simulink model "sysgenADCDAC"  (Simulink 7.3)
settings: Solver=ode45  StartTime=0.0  StopTime=20000  RelTol=1e-3
PreLoadFcn:
  | xlrequire('PreLoadFcn')
values from neighbouring files (symbols this model uses):
  Fstm = 0    [sysgenADCDAC_PreLoadFcn.m]
libraries: xbsIndex_r4 x94, xbsCopyrightNotice_r4 x1
settings Model: Creator=alexc  LastModifiedBy=douangp
settings DataIOCC: SignalLoggingName=sigsOut
settings OptimizationCC: BlockReduction=off  BooleanDataType=off  InlineInvariantSignals=on  InitFltsAndDblsToZero=on
settings DebuggingCC: SaveWithParameterizedLinksMsg=none  SignalResolutionControl=TryResolveAllWithWarning  SolverPrmCheckMsg=none  MultiTaskDSMMsg=warning  MultiTaskCondExecSysMsg=none  StrictBusMsg=None
settings HardwareCC: TargetUnknown=on
settings RTWCC: IncludeERTFirstTime=on
settings GRTTargetCC: TargetFcnLib=ansi_tfl_tmw.mat

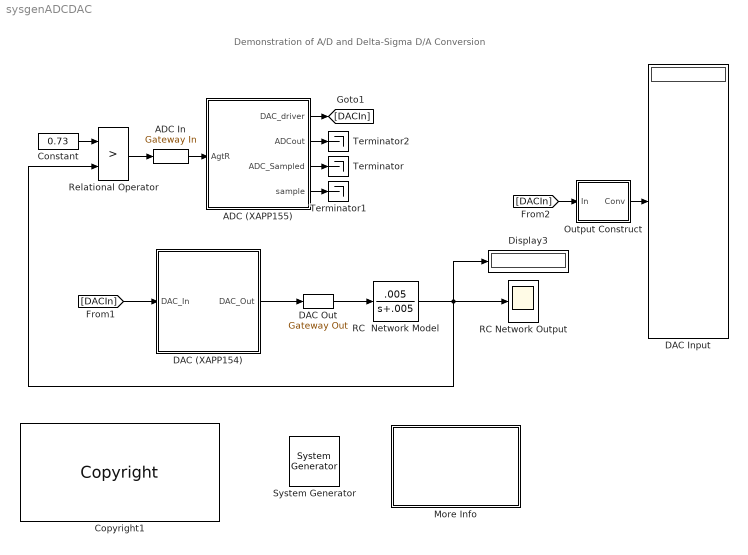
== system sysgenADCDAC ==
  note: Demonstration of A/D and Delta-Sigma D/A
      | Conversion
  " System Generator" : xbsIndex_r4/ System Generator  Tag=genX  SystemSampleTime=-1  xilinxfamily=virtex6  part=xc6vlx240t  speed=-1  package=ff1156  synthesis_tool=XST  clock_wrapper=Clock Enables  directory=./netlist  testbench=on  simulink_period=1  sysclk_period=2.5  dcm_input_clock_period=100  incr_netlist=off  trim_vbits=Everywhere in SubSystem  dbl_ovrd=According to Block Masks  core_generation=According to Block Masks  run_coregen=off  deprecated_control=off  eval_field=0  block_type=sysgen
      settings: block_version=9.2.00
  ADC (XAPP155) : Subsystem
  ADC In : xbsIndex_r4/Gateway In  arith_type=Unsigned  n_bits=1  bin_pt=0  quantization="Round  (unbiased: +/- Inf)"  overflow=Saturate  period=1  dbl_ovrd=off  timing_constraint=None  locs_specified=off  LOCs={}  block_type=gatewayin
      settings: infoedit="Gateway in block.  Converts inputs of type Simulink integer, double and fixed point to  Xilinx fixed point type.<P><P>Hardware notes:  In hardware these blocks become top level input ports."  xl_area=[0 0 0 0 1 0 0]  block_version=VER_STRING_GOES_HERE
  Constant : Constant  Value=0.73  OutDataType=sfix(16)  OutScaling=2^0
  Copyright1 : xbsCopyrightNotice_r4/Copyright  copyrighttext="Copyright (c) 2009  by  Xilinx, Inc. All rights reserved.<br><br>This file contains proprietary, confidential information of Xilinx, Inc., is distributed under licensefrom Xilinx, Inc., and may be used, copied and/or disclosed only pursuant to the terms of a valid licenseagreement with Xilinx, Inc. Xilinx hereby grants you a license to use this file solely for design,simulation, implementation and creation of design files limited to Xilinx devices or technologies. Use with non-Xilinx devices or technologies is expressly prohibited and immediately terminates your license unless covered by a separate agreement.<br><br>Xilinx is providing this design, code, or information \"as-is\" solely for use in developing programs and solutions for Xilinx devices, with no obligation on the part of Xilinx to provide support. By providingthis design, code, or information as one possible implementation of this feature, application or standard,Xilinx is making no representation that this implementation is free from any claims of infringement. Youare responsible for obtaining any rights you may require for your implementation. Xilinx expressly disclaimsany warranty whatsoever with respect to the adequacy of the implementation, including but not limited to anywarranties or representations that this implementation is free from claims of infringement, implied warrantiesof merchantability or fitness for a particular purpose.<br><br>Xilinx products are not intended for use in life support appliances, devices, or systems. Use in such applications is expressly prohibited.<br><br>Any modifications that are made to the Source Code are done at the user's sole risk and will be unsupported.<br><br>This copyright and support notice must be retained as part of this text at all times. (c) Copyright 1995-2009 Xilinx, Inc. All rights reserved."  block_type=copyright
      settings: block_version=10.1.00
      settings: infoedit=|
      | Copyright(C) 2008 by  Xilinx, Inc. All rights reserved.<br>
      | <br>
      | This file contains proprietary, confidential information of Xilinx, Inc., is distributed under license
      | from Xilinx, Inc., and may be used, copied and/or disclosed only pursuant to the terms of a valid license
      | agreement with Xilinx, Inc. Xilinx hereby grants you a license to use this file solely for design,
      | simulation, implementation and creation of design files limited to Xilinx devices or technologies. Use
      | with non-Xilinx devices or technologies is expressly prohibited and immediately terminates your license
      | unless covered by a separate agreement.<br>
      | <br>
      | Xilinx is providing this design, code, or information "as-is" solely for use in developing programs and
      | solutions for Xilinx devices, with no obligation on the part of Xilinx to provide support. By providing
      | this design, code, or information as one possible implementation of this feature, application or standard,
      | Xilinx is making no representation that this implementation is free from any claims of infringement. You
      | are responsible for obtaining any rights you may require for your implementation. Xilinx expressly disclaims
      | any warranty whatsoever with respect to the adequacy of the implementation, including but not limited to any
      | warranties or representations that this implementation is free from claims of infringement, implied warranties
      | of merchantability or fitness for a particular purpose.<br>
      | <br>
      | Xilinx products are not intended for use in life support appliances, devices, or systems. Use in such
      | applications is expressly prohibited.<br>
      | <br>
      | Any modifications that are made to the Source Code are done at the user's sole risk and will be unsupported.<br>
      | <br>
      | This copyright and support notice must be retained as part of this text at all times.
      | (c) Copyright 1995-2008 Xilinx, Inc. All rights reserved.
  DAC (XAPP154) : Subsystem
  DAC Input : Display
  DAC Out : xbsIndex_r4/Gateway Out  hdl_port=on  timing_constraint=None  locs_specified=off  LOCs={}  block_type=gatewayout
      settings: infoedit="Gateway out block.  Converts Xilinx fixed point inputs into ouputs of type Simulink integer, double, or fixed point.<P><P>Hardware notes:  In hardware these blocks become top level output ports or are discarded, depending on how they are configured."  xl_area=[0 0 0 0 1 0 0]  block_version=VER_STRING_GOES_HERE
  Display3 : Display
  More Info : Subsystem
      mask Display: disp('Double click\n for\n more information.')
  Output Construct : Subsystem
  RC  Network Model : TransferFcn  Numerator=[.005]  Denominator=[1 .005]
  "RC Network Output " : Scope
      settings: YMin=-0.1  YMax=1  MaxDataPoints=5000000
  Relational Operator : RelationalOperator  Operator=>  SampleTime=1  InputSameDT=on
  Terminator : Terminator
  Terminator1 : Terminator
  Terminator2 : Terminator
  wires:
  Relational Operator/1 -> ADC In/1
  Constant/1 -> Relational Operator/1
  ADC In/1 -> ADC (XAPP155)/1(AgtR)
  DAC (XAPP154)/1(DAC_Out) -> DAC Out/1
  DAC Out/1 -> RC  Network Model/1
  ADC (XAPP155)/2(ADCout) -> Terminator2/1
  ADC (XAPP155)/3(ADC_Sampled) -> Terminator/1
  ADC (XAPP155)/4(sample) -> Terminator1/1
  ADC (XAPP155)/1(DAC_driver) -> [DACIn]
  [DACIn] -> DAC (XAPP154)/1(DAC_In)
  RC  Network Model/1 -> Display3/1, Relational Operator/2, "RC Network Output "/1
  Output Construct/1(Conv) -> DAC Input/1
  [DACIn] -> Output Construct/1(In)

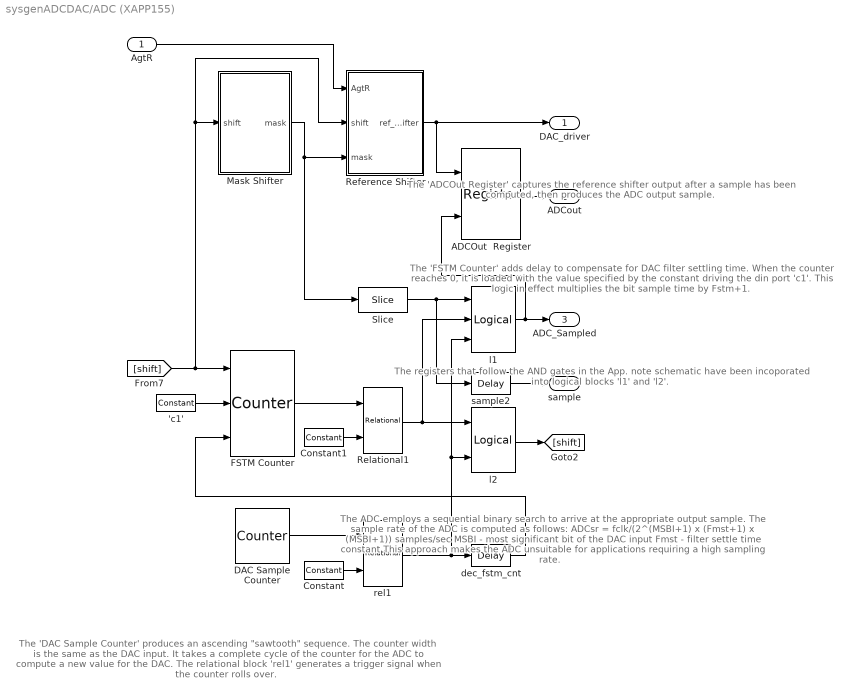
== system sysgenADCDAC/ADC (XAPP155) ==
  note: The 'DAC Sample Counter' produces an ascending
      | "sawtooth" sequence.  The counter width is the same
      | as the DAC input.  It takes a complete cycle of the
      | counter for the ADC to compute a new value for the DAC.
      | The relational block 'rel1' generates a trigger signal when
      |  the counter rolls over.
  note: The registers that follow the AND gates
      | in the App. note schematic have been
      | incoporated into logical blocks 'l1' and 'l2'.
  note: The ADC employs a sequential binary search to arrive at the
      | appropriate output sample.  The sample rate of the ADC is
      | computed as follows:
      |
      | ADCsr = fclk/(2^(MSBI+1) x (Fmst+1) x (MSBI+1)) samples/sec
      |
      | MSBI -  most significant bit of the DAC input
      | Fmst - filter settle time constant
      |
      | This approach makes the ADC unsuitable for applications
      |  requiring a high sampling rate.
  note: The 'ADCOut Register' captures the reference shifter
      | output after a sample has been computed, then produces the
      | ADC output sample.
  note: The 'FSTM Counter' adds delay to compensate for DAC
      | filter settling time.  When the counter reaches 0, it is
      | loaded with the value specified by the constant driving
      | the din port 'c1'.  This logic in effect multiplies the bit
      | sample time by Fstm+1.
  AgtR : Inport  OutDataType=sfix(16)  OutScaling=2^0
  'c1' : xbsIndex_r4/Constant  arith_type=Unsigned  const=Fstm  n_bits=4  bin_pt=0  explicit_period=off  period=1  equ=P=C  opselect=C  inp2=PCIN>>17  opr=+  inp1=P  carry=CIN  dbl_ovrd=off  block_type=constant
      settings: block_version=VER_STRING_GOES_HERE
  ADCOut  Register : xbsIndex_r4/Register  init=0  rst=off  en=on  dbl_ovrd=off  block_type=register
      settings: xl_area=[7 14 0 0 0 0 0]  block_version=VER_STRING_GOES_HERE
  Constant : xbsIndex_r4/Constant  arith_type=Unsigned  const=0  n_bits=14  bin_pt=0  explicit_period=off  period=1  equ=P=C  opselect=C  inp2=PCIN>>17  opr=+  inp1=P  carry=CIN  dbl_ovrd=off  block_type=constant
      settings: block_version=VER_STRING_GOES_HERE
  Constant1 : xbsIndex_r4/Constant  arith_type=Unsigned  const=0  n_bits=1  bin_pt=0  explicit_period=off  period=1  equ=P=C  opselect=C  inp2=PCIN>>17  opr=+  inp1=P  carry=CIN  dbl_ovrd=off  block_type=constant
      settings: block_version=VER_STRING_GOES_HERE
  DAC Sample Counter : xbsIndex_r4/Counter  cnt_type=Count Limited  cnt_to=Inf  operation=Up  start_count=0  cnt_by_val=1  arith_type=Unsigned  n_bits=10  bin_pt=0  load_pin=off  rst=off  en=off  explicit_period=off  period=1  dbl_ovrd=off  use_behavioral_HDL=off  implementation=Fabric  use_rpm=off  block_type=counter
      settings: infoedit="Configurable up, down and up/down counter.<P><P>Hardware notes: Free running counters are the least expensive in hardware.  A count limited counter is implemented by combining a counter with a comparator."  xl_area=[7 10 0 13 0 0 0]  block_version=VER_STRING_GOES_HERE
  FSTM Counter : xbsIndex_r4/Counter  cnt_type=Free Running  cnt_to=Inf  operation=Down  start_count=2  cnt_by_val=1  arith_type=Unsigned  n_bits=4  bin_pt=0  load_pin=on  rst=off  en=on  explicit_period=on  period=1  dbl_ovrd=off  use_behavioral_HDL=off  implementation=Fabric  use_rpm=off  block_type=counter
      settings: infoedit="Configurable up, down and up/down counter.<P><P>Hardware notes: Free running counters are the least expensive in hardware.  A count limited counter is implemented by combining a counter with a comparator."  xl_area=[4 4 0 5 0 0 0]  block_version=VER_STRING_GOES_HERE
  Mask Shifter : Subsystem
  "Reference Shifter " : Subsystem
  Relational1 : xbsIndex_r4/Relational  mode=a=b  en=off  latency=0  dbl_ovrd=off  block_type=relational
      settings: xl_area=[1 0 0 2 0 0 0]  block_version=VER_STRING_GOES_HERE
  Slice : xbsIndex_r4/Slice  nbits=1  boolean_output=on  mode=Lower Bit Location + Width  bit1=0  base1=MSB of Input  bit0=0  base0=LSB of Input  dbl_ovrd=off  block_type=slice
      settings: infoedit="Extracts a given range of bits from each input sample and presents it at the output.  The output type is ordinarily unsigned with binary point at zero, but can be Boolean when the slice is one bit wide.<P><P>Hardware notes: In hardware this block costs nothing."  block_version=VER_STRING_GOES_HERE
  dec_fstm_cnt : xbsIndex_r4/Delay  en=off  latency=1  dbl_ovrd=off  reg_retiming=off  block_type=delay
      settings: infoedit="Delay line having  configurable length.<P><P>Hardware notes: A delay line is a chain, each link of which is an SRL16 followed by a flip-flop. If register retiming is enabled, the delay line is a chain of flip-flops."  xl_area=[1 1 0 0 0 0 0]  block_version=VER_STRING_GOES_HERE
  l1 : xbsIndex_r4/Logical  logical_function=AND  inputs=3  en=off  latency=1  precision=Full  arith_type=Unsigned  n_bits=8  bin_pt=2  align_bp=on  dbl_ovrd=off  block_type=logical
      settings: xl_area=[1 1 0 1 0 0 0]  block_version=VER_STRING_GOES_HERE
  l2 : xbsIndex_r4/Logical  logical_function=AND  inputs=2  en=off  latency=1  precision=Full  arith_type=Unsigned  n_bits=8  bin_pt=2  align_bp=on  dbl_ovrd=off  block_type=logical
      settings: xl_area=[1 1 0 1 0 0 0]  block_version=VER_STRING_GOES_HERE
  rel1 : xbsIndex_r4/Relational  mode=a=b  en=off  latency=1  dbl_ovrd=off  block_type=relational
      settings: xl_area=[4 1 0 7 0 0 0]  block_version=VER_STRING_GOES_HERE
  sample2 : xbsIndex_r4/Delay  en=off  latency=1  dbl_ovrd=off  reg_retiming=off  block_type=delay
      settings: infoedit="Delay line having  configurable length.<P><P>Hardware notes: A delay line is a chain, each link of which is an SRL16 followed by a flip-flop. If register retiming is enabled, the delay line is a chain of flip-flops."  xl_area=[1 1 0 0 0 0 0]  block_version=VER_STRING_GOES_HERE
  DAC_driver : Outport  OutDataType=sfix(16)  OutScaling=2^0
  ADCout : Outport  Port=2  OutDataType=sfix(16)  OutScaling=2^0
  ADC_Sampled : Outport  Port=3  OutDataType=sfix(16)  OutScaling=2^0
  sample : Outport  Port=4  OutDataType=sfix(16)  OutScaling=2^0
  wires:
  Constant/1 -> rel1/2
  DAC Sample Counter/1 -> rel1/1
  sample2/1 -> sample/1
  l1/1 -> ADC_Sampled/1, ADCOut  Register/2
  Constant1/1 -> Relational1/2
  'c1'/1 -> FSTM Counter/2
  FSTM Counter/1 -> Relational1/1
  dec_fstm_cnt/1 -> FSTM Counter/3
  Mask Shifter/1(mask) -> Slice/1, "Reference Shifter "/3(mask)
  "Reference Shifter "/1(ref_shifter) -> DAC_driver/1, ADCOut  Register/1
  AgtR/1 -> "Reference Shifter "/1(AgtR)
  Slice/1 -> l1/1, sample2/1
  rel1/1 -> l2/2, l1/3, dec_fstm_cnt/1
  Relational1/1 -> l2/1, l1/2
  l2/1 -> [shift]
  [shift] -> Mask Shifter/1(shift), "Reference Shifter "/2(shift), FSTM Counter/1
  ADCOut  Register/1 -> ADCout/1

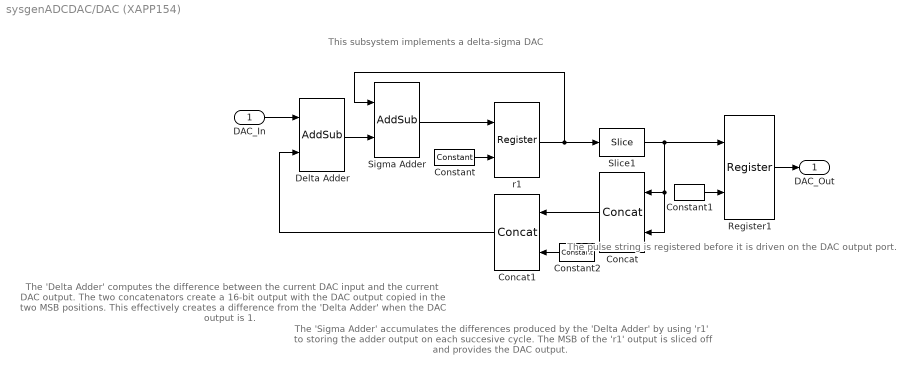
== system sysgenADCDAC/DAC (XAPP154) ==
  note: This subsystem implements a delta-sigma DAC
  note: The 'Delta Adder' computes the difference
      | between the current DAC input and the current
      | DAC output.  The two concatenators create
      | a 16-bit output with the DAC output copied in the
      | two MSB positions. This effectively creates a
      | difference from the 'Delta Adder' when the DAC
      | output is 1.
  note: The 'Sigma Adder' accumulates the
      | differences produced by the 'Delta Adder'
      | by using 'r1' to storing the adder output on
      | each succesive cycle.  The MSB of the 'r1'
      | output is sliced off and provides the DAC
      | output.
  note: The pulse string is registered before
      | it is driven on the DAC output port.
  DAC_In : Inport  OutDataType=sfix(16)  OutScaling=2^0
  Concat : xbsIndex_r4/Concat  num_inputs=2  dbl_ovrd=off  block_type=concat
      settings: block_version=VER_STRING_GOES_HERE
  Concat1 : xbsIndex_r4/Concat  num_inputs=2  dbl_ovrd=off  block_type=concat
      settings: block_version=VER_STRING_GOES_HERE
  Constant : xbsIndex_r4/Constant  arith_type=Boolean  const=0  n_bits=1  bin_pt=0  explicit_period=on  period=1  equ=P=C  opselect=C  inp2=PCIN>>17  opr=+  inp1=P  carry=CIN  dbl_ovrd=off  block_type=constant
      settings: block_version=VER_STRING_GOES_HERE
  Constant1 : xbsIndex_r4/Constant  arith_type=Boolean  const=0  n_bits=1  bin_pt=0  explicit_period=on  period=1  equ=P=C  opselect=C  inp2=PCIN>>17  opr=+  inp1=P  carry=CIN  dbl_ovrd=off  block_type=constant
      settings: block_version=VER_STRING_GOES_HERE
  Constant2 : xbsIndex_r4/Constant  arith_type=Unsigned  const=0  n_bits=14  bin_pt=0  explicit_period=on  period=1  equ=P=C  opselect=C  inp2=PCIN>>17  opr=+  inp1=P  carry=CIN  dbl_ovrd=off  block_type=constant
      settings: block_version=VER_STRING_GOES_HERE
  Delta Adder : xbsIndex_r4/AddSub  mode=Addition  use_carryin=off  use_carryout=off  en=off  latency=0  precision=User Defined  arith_type=Unsigned  n_bits=16  bin_pt=0  quantization=Truncate  overflow=Wrap  dbl_ovrd=off  use_behavioral_HDL=on  hw_selection=Fabric  pipelined=off  use_rpm=off  block_type=addsub
      settings: xl_area=[8 0 0 16 0 0 0]  block_version=VER_STRING_GOES_HERE
  Register1 : xbsIndex_r4/Register  init=0  rst=on  en=off  dbl_ovrd=off  block_type=register
      settings: xl_area=[1 1 0 0 0 0 0]  block_version=VER_STRING_GOES_HERE
  Sigma Adder : xbsIndex_r4/AddSub  mode=Addition  use_carryin=off  use_carryout=off  en=off  latency=0  precision=User Defined  arith_type=Unsigned  n_bits=16  bin_pt=0  quantization=Truncate  overflow=Wrap  dbl_ovrd=off  use_behavioral_HDL=on  hw_selection=Fabric  pipelined=off  use_rpm=off  block_type=addsub
      settings: xl_area=[8 0 0 16 0 0 0]  block_version=VER_STRING_GOES_HERE
  Slice1 : xbsIndex_r4/Slice  nbits=1  boolean_output=off  mode=Upper Bit Location + Width  bit1=0  base1=MSB of Input  bit0=0  base0=LSB of Input  dbl_ovrd=off  block_type=slice
      settings: infoedit="Extracts a given range of bits from each input sample and presents it at the output.  The output type is ordinarily unsigned with binary point at zero, but can be Boolean when the slice is one bit wide.<P><P>Hardware notes: In hardware this block costs nothing."  block_version=VER_STRING_GOES_HERE
  r1 : xbsIndex_r4/Register  init=2^6  rst=on  en=off  dbl_ovrd=off  block_type=register
      settings: xl_area=[8 16 0 0 0 0 0]  block_version=VER_STRING_GOES_HERE
  DAC_Out : Outport  OutDataType=sfix(16)  OutScaling=2^0
  wires:
  DAC_In/1 -> Delta Adder/1
  Register1/1 -> DAC_Out/1
  r1/1 -> Slice1/1, Sigma Adder/1
  Sigma Adder/1 -> r1/1
  Constant/1 -> r1/2
  Concat1/1 -> Delta Adder/2
  Concat/1 -> Concat1/1
  Slice1/1 -> Register1/1, Concat/1, Concat/2
  Constant2/1 -> Concat1/2
  Constant1/1 -> Register1/2
  Delta Adder/1 -> Sigma Adder/2

== system sysgenADCDAC/More Info ==
  note: Demonstration of A/D and Delta-Sigma D/A Conversion
  note: This model implements a 14-bit analog to digital converter (ADC) and a digital to analog converter
      | (DAC) for Virtex and Virtex derivative devices.  The model is based on the delta-sigma DAC and ADC
      | implementations described, respectively, in Xilinx App. Notes 154 and 155 by John Logue.  Both
      | documents can be found at
      |
      |   http://www.xilinx.com/apps/appsweb.htm
      |
      | The ADC requires feedback from the DAC to compute output samples.  The DAC output is a pulse
      | string whose duty cycle is proportional to the amplitude of the desired output voltage.  XAPP154
      | describes a low-pass filter on the DAC output implemented with an RC network.  Here the RC network
      | is simulated using a transfer function block.  XAPP155 specifies an op-amp circuit on the input of
      | the ADC.  In this model, the op-amp is replaced by a relational block.
      |
      | When simulating this model, the behavior is best viewed with the simulation duration set to Inf.  The
      | DAC input display shows the a binary representation of the DAC input and illustrates the binary search
      | used by the ADC to constructs a digital sample of the input voltage (in this case .73).
      |
      | This design occupies 54 Slice LUTs (1%), 62 Slice Registers (1%) of an xc6vlx240t-1ff1156 part
      | and runs over 400 MHz.

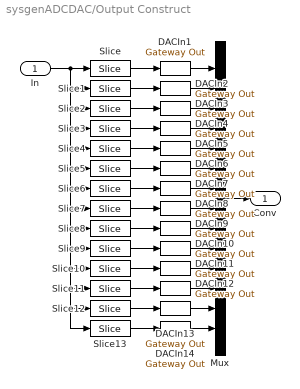
== system sysgenADCDAC/Output Construct ==
  In : Inport  OutDataType=sfix(16)  OutScaling=2^0
  DACIn{1..14} (14 alike) : xbsIndex_r4/Gateway Out  hdl_port=off  timing_constraint=None  locs_specified=off  LOCs={}  block_type=gatewayout
      settings: infoedit="Gateway out block.  Converts Xilinx fixed point inputs into ouputs of type Simulink integer, double, or fixed point.<P><P>Hardware notes:  In hardware these blocks become top level output ports or are discarded, depending on how they are configured."  xl_area=[0 0 0 0 0 0 0]  block_version=VER_STRING_GOES_HERE
  Mux : Mux  Inputs=14
  Slice : xbsIndex_r4/Slice  nbits=1  boolean_output=off  mode=Lower Bit Location + Width  bit1=0  base1=MSB of Input  bit0=13  base0=LSB of Input  dbl_ovrd=off  block_type=slice
      settings: infoedit="Extracts a given range of bits from each input sample and presents it at the output.  The output type is ordinarily unsigned with binary point at zero, but can be Boolean when the slice is one bit wide.<P><P>Hardware notes: In hardware this block costs nothing."  block_version=VER_STRING_GOES_HERE
  Slice1 : xbsIndex_r4/Slice  nbits=1  boolean_output=off  mode=Lower Bit Location + Width  bit1=0  base1=MSB of Input  bit0=12  base0=LSB of Input  dbl_ovrd=off  block_type=slice
      settings: infoedit="Extracts a given range of bits from each input sample and presents it at the output.  The output type is ordinarily unsigned with binary point at zero, but can be Boolean when the slice is one bit wide.<P><P>Hardware notes: In hardware this block costs nothing."  block_version=VER_STRING_GOES_HERE
  Slice10 : xbsIndex_r4/Slice  nbits=1  boolean_output=off  mode=Lower Bit Location + Width  bit1=0  base1=MSB of Input  bit0=3  base0=LSB of Input  dbl_ovrd=off  block_type=slice
      settings: infoedit="Extracts a given range of bits from each input sample and presents it at the output.  The output type is ordinarily unsigned with binary point at zero, but can be Boolean when the slice is one bit wide.<P><P>Hardware notes: In hardware this block costs nothing."  block_version=VER_STRING_GOES_HERE
  Slice11 : xbsIndex_r4/Slice  nbits=1  boolean_output=off  mode=Lower Bit Location + Width  bit1=0  base1=MSB of Input  bit0=2  base0=LSB of Input  dbl_ovrd=off  block_type=slice
      settings: infoedit="Extracts a given range of bits from each input sample and presents it at the output.  The output type is ordinarily unsigned with binary point at zero, but can be Boolean when the slice is one bit wide.<P><P>Hardware notes: In hardware this block costs nothing."  block_version=VER_STRING_GOES_HERE
  Slice12 : xbsIndex_r4/Slice  nbits=1  boolean_output=off  mode=Lower Bit Location + Width  bit1=0  base1=MSB of Input  bit0=1  base0=LSB of Input  dbl_ovrd=off  block_type=slice
      settings: infoedit="Extracts a given range of bits from each input sample and presents it at the output.  The output type is ordinarily unsigned with binary point at zero, but can be Boolean when the slice is one bit wide.<P><P>Hardware notes: In hardware this block costs nothing."  block_version=VER_STRING_GOES_HERE
  Slice13 : xbsIndex_r4/Slice  nbits=1  boolean_output=off  mode=Lower Bit Location + Width  bit1=0  base1=MSB of Input  bit0=0  base0=LSB of Input  dbl_ovrd=off  block_type=slice
      settings: infoedit="Extracts a given range of bits from each input sample and presents it at the output.  The output type is ordinarily unsigned with binary point at zero, but can be Boolean when the slice is one bit wide.<P><P>Hardware notes: In hardware this block costs nothing."  block_version=VER_STRING_GOES_HERE
  Slice2 : xbsIndex_r4/Slice  nbits=1  boolean_output=off  mode=Lower Bit Location + Width  bit1=0  base1=MSB of Input  bit0=11  base0=LSB of Input  dbl_ovrd=off  block_type=slice
      settings: infoedit="Extracts a given range of bits from each input sample and presents it at the output.  The output type is ordinarily unsigned with binary point at zero, but can be Boolean when the slice is one bit wide.<P><P>Hardware notes: In hardware this block costs nothing."  block_version=VER_STRING_GOES_HERE
  Slice3 : xbsIndex_r4/Slice  nbits=1  boolean_output=off  mode=Lower Bit Location + Width  bit1=0  base1=MSB of Input  bit0=10  base0=LSB of Input  dbl_ovrd=off  block_type=slice
      settings: infoedit="Extracts a given range of bits from each input sample and presents it at the output.  The output type is ordinarily unsigned with binary point at zero, but can be Boolean when the slice is one bit wide.<P><P>Hardware notes: In hardware this block costs nothing."  block_version=VER_STRING_GOES_HERE
  Slice4 : xbsIndex_r4/Slice  nbits=1  boolean_output=off  mode=Lower Bit Location + Width  bit1=0  base1=MSB of Input  bit0=9  base0=LSB of Input  dbl_ovrd=off  block_type=slice
      settings: infoedit="Extracts a given range of bits from each input sample and presents it at the output.  The output type is ordinarily unsigned with binary point at zero, but can be Boolean when the slice is one bit wide.<P><P>Hardware notes: In hardware this block costs nothing."  block_version=VER_STRING_GOES_HERE
  Slice5 : xbsIndex_r4/Slice  nbits=1  boolean_output=off  mode=Lower Bit Location + Width  bit1=0  base1=MSB of Input  bit0=8  base0=LSB of Input  dbl_ovrd=off  block_type=slice
      settings: infoedit="Extracts a given range of bits from each input sample and presents it at the output.  The output type is ordinarily unsigned with binary point at zero, but can be Boolean when the slice is one bit wide.<P><P>Hardware notes: In hardware this block costs nothing."  block_version=VER_STRING_GOES_HERE
  Slice6 : xbsIndex_r4/Slice  nbits=1  boolean_output=off  mode=Lower Bit Location + Width  bit1=0  base1=MSB of Input  bit0=7  base0=LSB of Input  dbl_ovrd=off  block_type=slice
      settings: infoedit="Extracts a given range of bits from each input sample and presents it at the output.  The output type is ordinarily unsigned with binary point at zero, but can be Boolean when the slice is one bit wide.<P><P>Hardware notes: In hardware this block costs nothing."  block_version=VER_STRING_GOES_HERE
  Slice7 : xbsIndex_r4/Slice  nbits=1  boolean_output=off  mode=Lower Bit Location + Width  bit1=0  base1=MSB of Input  bit0=6  base0=LSB of Input  dbl_ovrd=off  block_type=slice
      settings: infoedit="Extracts a given range of bits from each input sample and presents it at the output.  The output type is ordinarily unsigned with binary point at zero, but can be Boolean when the slice is one bit wide.<P><P>Hardware notes: In hardware this block costs nothing."  block_version=VER_STRING_GOES_HERE
  Slice8 : xbsIndex_r4/Slice  nbits=1  boolean_output=off  mode=Lower Bit Location + Width  bit1=0  base1=MSB of Input  bit0=5  base0=LSB of Input  dbl_ovrd=off  block_type=slice
      settings: infoedit="Extracts a given range of bits from each input sample and presents it at the output.  The output type is ordinarily unsigned with binary point at zero, but can be Boolean when the slice is one bit wide.<P><P>Hardware notes: In hardware this block costs nothing."  block_version=VER_STRING_GOES_HERE
  Slice9 : xbsIndex_r4/Slice  nbits=1  boolean_output=off  mode=Lower Bit Location + Width  bit1=0  base1=MSB of Input  bit0=4  base0=LSB of Input  dbl_ovrd=off  block_type=slice
      settings: infoedit="Extracts a given range of bits from each input sample and presents it at the output.  The output type is ordinarily unsigned with binary point at zero, but can be Boolean when the slice is one bit wide.<P><P>Hardware notes: In hardware this block costs nothing."  block_version=VER_STRING_GOES_HERE
  Conv : Outport  OutDataType=sfix(16)  OutScaling=2^0
  wires:
  In/1 -> Slice13/1, Slice12/1, Slice11/1, Slice10/1, Slice9/1, Slice8/1, Slice7/1, Slice6/1, Slice5/1, Slice4/1, Slice3/1, Slice2/1, Slice1/1, Slice/1
  Slice/1 -> DACIn1/1
  Slice1/1 -> DACIn2/1
  Slice2/1 -> DACIn3/1
  Slice3/1 -> DACIn4/1
  Slice4/1 -> DACIn5/1
  Slice5/1 -> DACIn6/1
  Slice6/1 -> DACIn7/1
  Slice7/1 -> DACIn8/1
  Slice8/1 -> DACIn9/1
  Slice9/1 -> DACIn10/1
  Slice10/1 -> DACIn11/1
  Slice11/1 -> DACIn12/1
  Slice12/1 -> DACIn13/1
  Slice13/1 -> DACIn14/1
  DACIn1/1 -> Mux/1
  DACIn2/1 -> Mux/2
  DACIn3/1 -> Mux/3
  DACIn4/1 -> Mux/4
  DACIn5/1 -> Mux/5
  DACIn6/1 -> Mux/6
  DACIn7/1 -> Mux/7
  DACIn8/1 -> Mux/8
  DACIn9/1 -> Mux/9
  DACIn10/1 -> Mux/10
  DACIn11/1 -> Mux/11
  DACIn12/1 -> Mux/12
  DACIn13/1 -> Mux/13
  DACIn14/1 -> Mux/14
  Mux/1 -> Conv/1

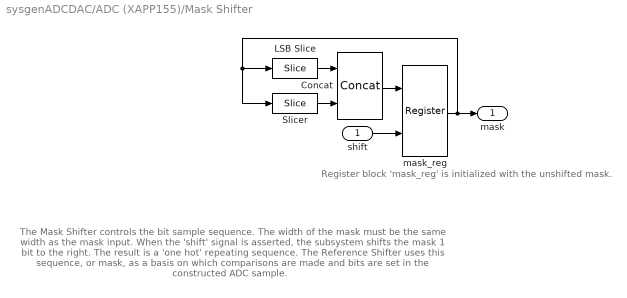
== system sysgenADCDAC/ADC (XAPP155)/Mask Shifter ==
  note: The Mask Shifter controls the bit sample sequence.  The width
      | of the mask must be the same width as the mask input.  When
      | the 'shift' signal is asserted, the subsystem shifts the mask 1
      | bit to the right.  The result is a 'one hot' repeating sequence.
      | The Reference Shifter uses this sequence, or mask, as a basis
      | on which comparisons are made and bits are set in the
      | constructed ADC sample.
  note: Register block 'mask_reg' is initialized
      | with the unshifted mask.
  shift : Inport  OutDataType=sfix(16)  OutScaling=2^0
  Concat : xbsIndex_r4/Concat  num_inputs=2  dbl_ovrd=off  block_type=concat
      settings: block_version=VER_STRING_GOES_HERE
  LSB Slice : xbsIndex_r4/Slice  nbits=1  boolean_output=off  mode=Lower Bit Location + Width  bit1=0  base1=MSB of Input  bit0=0  base0=LSB of Input  dbl_ovrd=off  block_type=slice
      settings: infoedit="Extracts a given range of bits from each input sample and presents it at the output.  The output type is ordinarily unsigned with binary point at zero, but can be Boolean when the slice is one bit wide.<P><P>Hardware notes: In hardware this block costs nothing."  block_version=VER_STRING_GOES_HERE
  Slicer : xbsIndex_r4/Slice  nbits=13  boolean_output=off  mode=Upper Bit Location + Width  bit1=0  base1=MSB of Input  bit0=0  base0=LSB of Input  dbl_ovrd=off  block_type=slice
      settings: infoedit="Extracts a given range of bits from each input sample and presents it at the output.  The output type is ordinarily unsigned with binary point at zero, but can be Boolean when the slice is one bit wide.<P><P>Hardware notes: In hardware this block costs nothing."  block_version=VER_STRING_GOES_HERE
  mask_reg : xbsIndex_r4/Register  init=2^13  rst=off  en=on  dbl_ovrd=off  block_type=register
      settings: xl_area=[7 14 0 0 0 0 0]  block_version=VER_STRING_GOES_HERE
  mask : Outport  OutDataType=sfix(16)  OutScaling=2^0
  wires:
  Concat/1 -> mask_reg/1
  Slicer/1 -> Concat/2
  LSB Slice/1 -> Concat/1
  shift/1 -> mask_reg/2
  mask_reg/1 -> mask/1, LSB Slice/1, Slicer/1

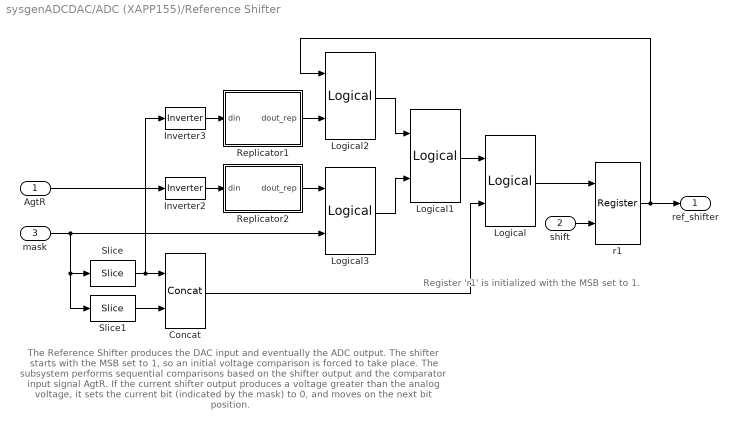
== system sysgenADCDAC/ADC (XAPP155)/Reference Shifter  ==
  note: The Reference Shifter produces the DAC input and eventually the
      | ADC output.  The shifter starts with the MSB set to 1, so an
      | initial voltage comparison is forced to take place.
      |
      | The subsystem performs sequential comparisons based on the
      | shifter output and the comparator input signal AgtR.  If the current
      | shifter output produces a voltage greater than the analog voltage,
      | it sets the current bit (indicated by the mask) to 0, and moves on
      | the next bit position.
  note: Register 'r1' is initialized with the MSB
      | set to 1.
  AgtR : Inport  OutDataType=sfix(16)  OutScaling=2^0
  shift : Inport  Port=2  OutDataType=sfix(16)  OutScaling=2^0
  mask : Inport  Port=3  OutDataType=sfix(16)  OutScaling=2^0
  Concat : xbsIndex_r4/Concat  num_inputs=2  dbl_ovrd=off  block_type=concat
      settings: block_version=VER_STRING_GOES_HERE
  Inverter2 : xbsIndex_r4/Inverter  en=off  latency=0  dbl_ovrd=off  block_type=inv
      settings: xl_area=[0 0 0 0 0 0 0]  block_version=VER_STRING_GOES_HERE
  Inverter3 : xbsIndex_r4/Inverter  en=off  latency=0  dbl_ovrd=off  block_type=inv
      settings: xl_area=[0 0 0 0 0 0 0]  block_version=VER_STRING_GOES_HERE
  Logical : xbsIndex_r4/Logical  logical_function=OR  inputs=2  en=off  latency=0  precision=User Defined  arith_type=Unsigned  n_bits=14  bin_pt=0  align_bp=on  dbl_ovrd=off  block_type=logical
      settings: xl_area=[14 0 0 14 0 0 0]  block_version=VER_STRING_GOES_HERE
  Logical1 : xbsIndex_r4/Logical  logical_function=AND  inputs=2  en=off  latency=0  precision=User Defined  arith_type=Unsigned  n_bits=14  bin_pt=0  align_bp=on  dbl_ovrd=off  block_type=logical
      settings: xl_area=[14 0 0 14 0 0 0]  block_version=VER_STRING_GOES_HERE
  Logical2 : xbsIndex_r4/Logical  logical_function=AND  inputs=2  en=off  latency=0  precision=User Defined  arith_type=Unsigned  n_bits=14  bin_pt=0  align_bp=on  dbl_ovrd=off  block_type=logical
      settings: xl_area=[14 0 0 14 0 0 0]  block_version=VER_STRING_GOES_HERE
  Logical3 : xbsIndex_r4/Logical  logical_function=NAND  inputs=2  en=off  latency=0  precision=User Defined  arith_type=Unsigned  n_bits=14  bin_pt=0  align_bp=on  dbl_ovrd=off  block_type=logical
      settings: xl_area=[14 0 0 14 0 0 0]  block_version=VER_STRING_GOES_HERE
  Replicator1 : Subsystem
  Replicator2 : Subsystem
  Slice : xbsIndex_r4/Slice  nbits=1  boolean_output=off  mode=Lower Bit Location + Width  bit1=0  base1=MSB of Input  bit0=0  base0=LSB of Input  dbl_ovrd=off  block_type=slice
      settings: infoedit="Extracts a given range of bits from each input sample and presents it at the output.  The output type is ordinarily unsigned with binary point at zero, but can be Boolean when the slice is one bit wide.<P><P>Hardware notes: In hardware this block costs nothing."  block_version=VER_STRING_GOES_HERE
  Slice1 : xbsIndex_r4/Slice  nbits=13  boolean_output=off  mode=Upper Bit Location + Width  bit1=0  base1=MSB of Input  bit0=0  base0=LSB of Input  dbl_ovrd=off  block_type=slice
      settings: infoedit="Extracts a given range of bits from each input sample and presents it at the output.  The output type is ordinarily unsigned with binary point at zero, but can be Boolean when the slice is one bit wide.<P><P>Hardware notes: In hardware this block costs nothing."  block_version=VER_STRING_GOES_HERE
  r1 : xbsIndex_r4/Register  init=2^13  rst=off  en=on  dbl_ovrd=off  block_type=register
      settings: xl_area=[7 14 0 0 0 0 0]  block_version=VER_STRING_GOES_HERE
  ref_shifter : Outport  OutDataType=sfix(16)  OutScaling=2^0
  wires:
  Logical/1 -> r1/1
  Logical1/1 -> Logical/1
  Logical2/1 -> Logical1/1
  Logical3/1 -> Logical1/2
  Slice/1 -> Inverter3/1, Concat/1
  Slice1/1 -> Concat/2
  mask/1 -> Slice/1, Slice1/1, Logical3/2
  Concat/1 -> Logical/2
  AgtR/1 -> Inverter2/1
  Replicator1/1(dout_rep) -> Logical2/2
  Replicator2/1(dout_rep) -> Logical3/1
  r1/1 -> ref_shifter/1, Logical2/1
  shift/1 -> r1/2
  Inverter3/1 -> Replicator1/1(din)
  Inverter2/1 -> Replicator2/1(din)

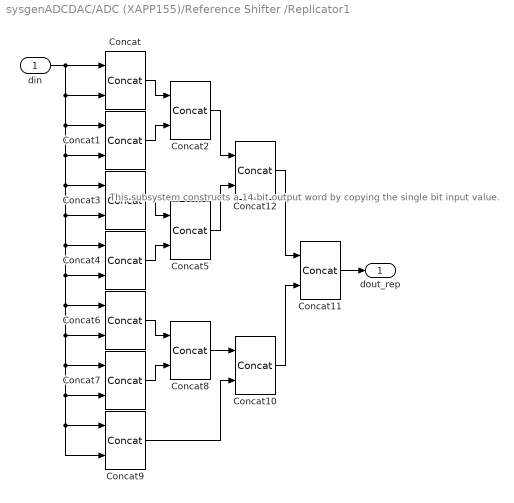
== system sysgenADCDAC/ADC (XAPP155)/Reference Shifter /Replicator1 ==
  note: This subsystem constructs a 14-bit output word
      | by copying the single bit input value.
  din : Inport  OutDataType=sfix(16)  OutScaling=2^0
  Concat{,1..12} (13 alike) : xbsIndex_r4/Concat  num_inputs=2  dbl_ovrd=off  block_type=concat
      settings: block_version=VER_STRING_GOES_HERE
  dout_rep : Outport  OutDataType=sfix(16)  OutScaling=2^0
  wires:
  Concat/1 -> Concat2/1
  Concat1/1 -> Concat2/2
  Concat3/1 -> Concat5/1
  Concat4/1 -> Concat5/2
  Concat6/1 -> Concat8/1
  Concat7/1 -> Concat8/2
  Concat9/1 -> Concat10/2
  Concat2/1 -> Concat12/1
  Concat5/1 -> Concat12/2
  Concat8/1 -> Concat10/1
  Concat12/1 -> Concat11/1
  Concat10/1 -> Concat11/2
  din/1 -> Concat/1, Concat/2, Concat9/2, Concat9/1, Concat7/2, Concat7/1, Concat6/2, Concat6/1, Concat4/2, Concat4/1, Concat3/2, Concat3/1, Concat1/2, Concat1/1
  Concat11/1 -> dout_rep/1

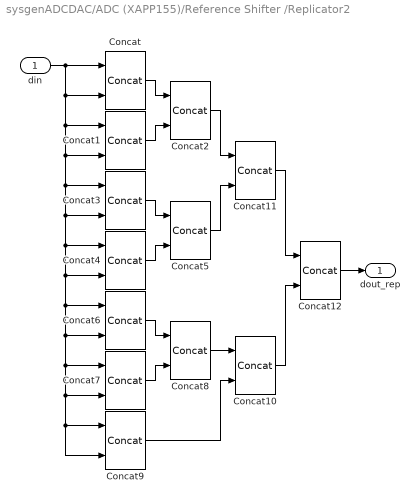
== system sysgenADCDAC/ADC (XAPP155)/Reference Shifter /Replicator2 ==
  din : Inport  OutDataType=sfix(16)  OutScaling=2^0
  Concat{,1..12} (13 alike) : xbsIndex_r4/Concat  num_inputs=2  dbl_ovrd=off  block_type=concat
      settings: block_version=VER_STRING_GOES_HERE
  dout_rep : Outport  OutDataType=sfix(16)  OutScaling=2^0
  wires:
  Concat/1 -> Concat2/1
  Concat1/1 -> Concat2/2
  Concat3/1 -> Concat5/1
  Concat4/1 -> Concat5/2
  Concat6/1 -> Concat8/1
  Concat7/1 -> Concat8/2
  Concat9/1 -> Concat10/2
  Concat2/1 -> Concat11/1
  Concat5/1 -> Concat11/2
  Concat8/1 -> Concat10/1
  Concat11/1 -> Concat12/1
  Concat10/1 -> Concat12/2
  din/1 -> Concat1/2, Concat3/1, Concat9/1, Concat9/2, Concat7/2, Concat7/1, Concat6/2, Concat6/1, Concat4/2, Concat4/1, Concat3/2, Concat1/1, Concat/2, Concat/1
  Concat12/1 -> dout_rep/1
